simulink model "trayectoria_odometria_switch"  (R2021b)
settings: Solver=VariableStepAuto  StartTime=0.0  StopTime=40  RelTol=1e-3
model workspace (MAT data in the model file):
  dg = 0.2
settings Model: Creator=Mauri  LastModifiedBy=Mauri

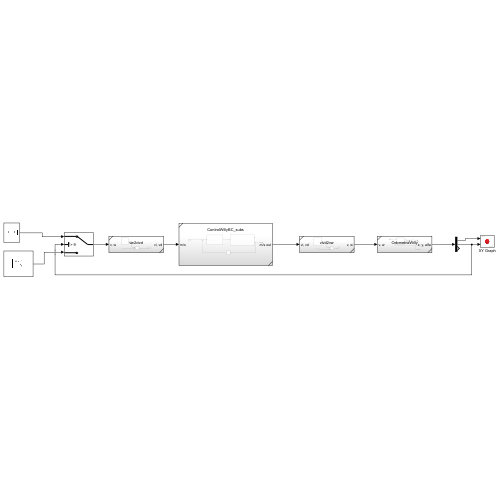
[thumbnail: Simulink's stored preview of the top-level diagram]
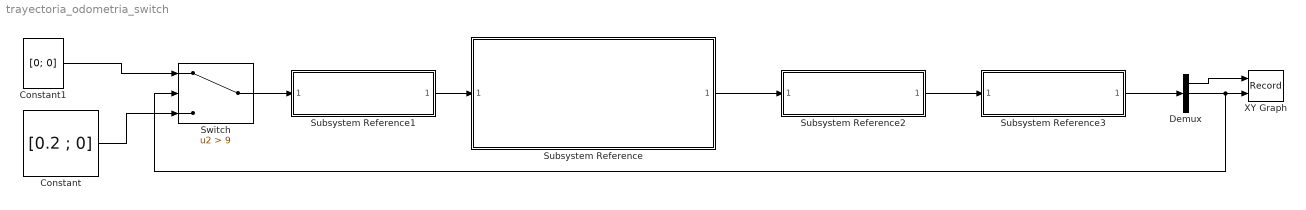
== system trayectoria_odometria_switch ==
  Constant : Constant  Value=[0.2 ; 0]  VectorParams1D=off  SampleTime=0.01
  Constant1 : Constant  Value=[0; 0]
  Demux : Demux  Outputs=3
  Subsystem Reference : Subsystem  ReferencedSubsystem=ControlWillyBC_subs
  Subsystem Reference1 : Subsystem  ReferencedSubsystem=vw2vivd
  Subsystem Reference2 : Subsystem  ReferencedSubsystem=vivd2vw
  Subsystem Reference3 : Subsystem  ReferencedSubsystem=OdometriaWilly
  Switch : Switch  Criteria=u2 > Threshold  Threshold=9
  XY Graph : Record  FileSettingsInternal="{\"entries\":[{\"content\":{\"excelSettings\":{\"content\":{},\"type\":\"Streamout.ExcelSettings\"}},\"type\":\"Streamout.FileSettingStorage\",\"uuid\":\"0cfdb027-3065-4385-a9cd-61346e31d7e2\"}],\"packageUris\":[\"http://schema.mathworks.com/mf0/streamout_blocks/R2020a\"],\"version\":\"1.0\"}"  Layout=[1 1]  SignalsInternal="{\"entries\":[{\"content\":{\"signals\":[{\"content\":{\"blockPath\":[\"untitled/XY Graph\"],\"channel\":[],\"dimensions\":[1],\"domain\":\"untitled/XY Graph\",\"lineColor\":\"#a2142f\",\"plots\":[1],\"port\":1,\"sid\":[\"\"],\"signalID\":1491,\"signalName\":\"Demux:1\"},\"type\":\"RecordBlkView.Signal\",\"uuid\":\"65c26113-44d4-4361-be2f-c78b75f787eb\"},{\"content\":{\"blockPath\":[\"untitled/XY Graph\"],\"channel\":[],\"dimensions\":[1],\"domain\":\"untitled/XY Graph\",\"lineColor\":\"#139fff\",\"plots\":[1],\"port\":2,\"sid\":[\"\"],\"signalID\":1495,\"signalName\":\"Demux:2\"},\"type\":\"RecordBlkView.Signal\",\"uuid\":\"11d5284b-700d-4888-b3ee-a669ab244c7f\"}]},\"type\":\"RecordBlkView.InputSignals\",\"uuid\":\"6930027e-80a0-47cb-aa3d-08d4e37a26d6\"}],\"packageUris\":[\"http://schema.mathworks.com/mf0/streamout_blocks/R2020a\"],\"version\":\"1.0\"}"  VisualizationBindings="{\"xyplotplugin\":{\"info\":[{\"series\":[{\"bindingParametersList\":[{\"parameter\":\"X-Axis\",\"signalID\":1491,\"signalName\":\"Demux:1\"},{\"parameter\":\"Y-Axis\",\"signalID\":1495,\"signalName\":\"Demux:2\"}],\"seriesID\":20406}],\"subplotID\":1}]}}"  CompatibilityTag=XY
  wires:
  Demux/2 -> XY Graph/2, Switch/2
  Demux/1 -> XY Graph/1
  Subsystem Reference/1 -> Subsystem Reference2/1
  Subsystem Reference3/1 -> Demux/1
  Subsystem Reference1/1 -> Subsystem Reference/1
  Subsystem Reference2/1 -> Subsystem Reference3/1
  Switch/1 -> Subsystem Reference1/1
  Constant1/1 -> Switch/1
  Constant/1 -> Switch/3
